simulink library "PQFV_lib"  (Simulink 8.1)
settings: Solver=ode45  StartTime=0.0  StopTime=10.0  RelTol=1e-3
undefined symbols (not defined in the file): Ts
libraries: powerlib_extras x6, RMS_lib x2
settings Model: Creator=RE25624  LastModifiedBy=g73labuser

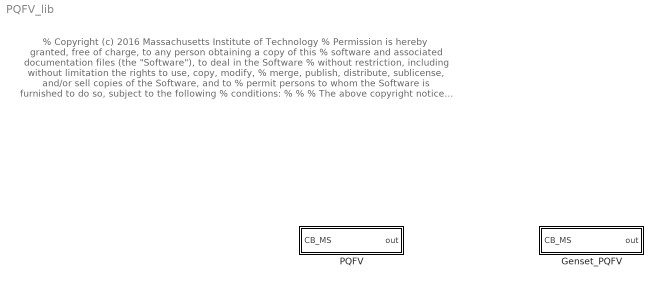
== system PQFV_lib ==
  note: % Copyright (c) 2016 Massachusetts Institute of Technology
      | % Permission is hereby granted, free of charge, to any person obtaining a copy of this
      | % software and associated documentation files (the "Software"), to deal in the Software
      | % without restriction, including without limitation the rights to use, copy, modify,
      | % merge, publish, distribute, sublicense, and/or sell copies of the Software, and to
      | % permit persons to whom the Software is furnished to do so, subject to the following
      | % conditions:
      | %
      | %
      | % The above copyright notice and this permission notice shall be included in
      | % all copies or substantial portions of the Software.
      | %
      | % THE SOFTWARE IS PROVIDED "AS IS", WITHOUT WARRANTY OF ANY KIND, EXPRESS OR IMPLIED,
      | % INCLUDING BUT NOT LIMITED TO THE WARRANTIES OF MERCHANTABILITY, FITNESS FOR A
      | % PARTICULAR PURPOSE AND NONINFRINGEMENT. IN NO EVENT SHALL THE AUTHORS OR COPYRIGHT
      | % HOLDERS BE LIABLE FOR ANY CLAIM, DAMAGES OR OTHER LIABILITY, WHETHER IN AN ACTION
      | % OF CONTRACT, TORT OR OTHERWISE, ARISING FROM, OUT OF OR IN CONNECTION WITH THE
      | % SOFTWARE OR THE USE OR OTHER DEALINGS IN THE SOFTWARE.
      | %
      | %
      | %%
  Genset_PQFV : Subsystem  mask(PQFV){VRMSLL=13800, Ts=Ts}
      mask prompts: VRMSLL "Nominal VRMSLL"; Ts "Sample Time [Sec]"
      mask help:
      | Block inputs: circuit breaker measurements
      | Block outputs: kW, kVAR, Hz, VRMSLL, Vpu, cb-status
      | -voltage as seem at the entry-point of the circuit breaker
  PQFV : Subsystem  mask(PQFV){VRMSLL=13800, Ts=Ts}
      mask prompts: VRMSLL "Nominal VRMSLL"; Ts "Sample Time [Sec]"
      mask help:
      | Block inputs: circuit breaker measurements
      | Block outputs: kW, kVAR, Hz, VRMSLL, Vpu, cb-status
      | -voltage as seem at the entry-point of the circuit breaker

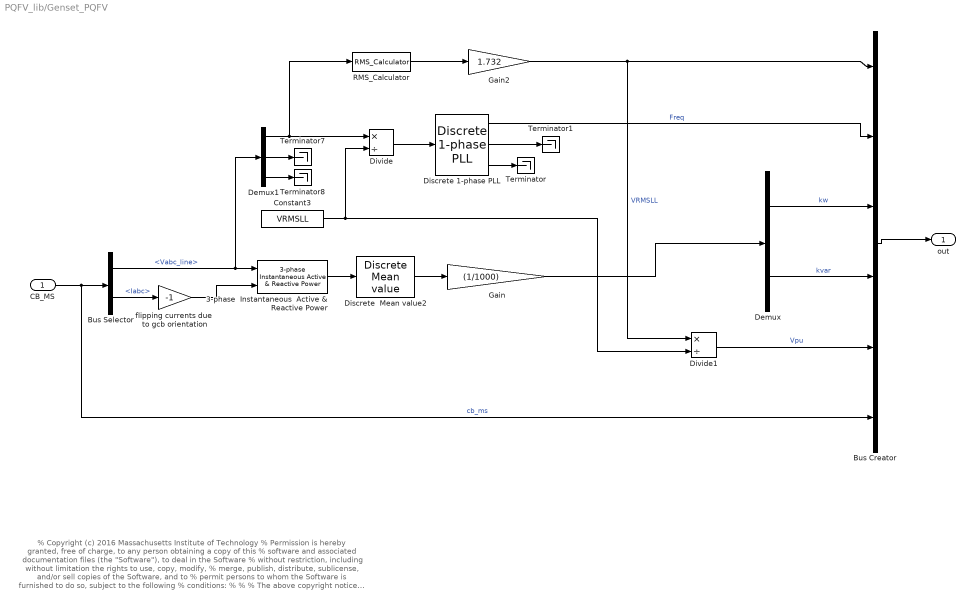
== system PQFV_lib/Genset_PQFV ==
  note: % Copyright (c) 2016 Massachusetts Institute of Technology
      | % Permission is hereby granted, free of charge, to any person obtaining a copy of this
      | % software and associated documentation files (the "Software"), to deal in the Software
      | % without restriction, including without limitation the rights to use, copy, modify,
      | % merge, publish, distribute, sublicense, and/or sell copies of the Software, and to
      | % permit persons to whom the Software is furnished to do so, subject to the following
      | % conditions:
      | %
      | %
      | % The above copyright notice and this permission notice shall be included in
      | % all copies or substantial portions of the Software.
      | %
      | % THE SOFTWARE IS PROVIDED "AS IS", WITHOUT WARRANTY OF ANY KIND, EXPRESS OR IMPLIED,
      | % INCLUDING BUT NOT LIMITED TO THE WARRANTIES OF MERCHANTABILITY, FITNESS FOR A
      | % PARTICULAR PURPOSE AND NONINFRINGEMENT. IN NO EVENT SHALL THE AUTHORS OR COPYRIGHT
      | % HOLDERS BE LIABLE FOR ANY CLAIM, DAMAGES OR OTHER LIABILITY, WHETHER IN AN ACTION
      | % OF CONTRACT, TORT OR OTHERWISE, ARISING FROM, OUT OF OR IN CONNECTION WITH THE
      | % SOFTWARE OR THE USE OR OTHER DEALINGS IN THE SOFTWARE.
      | %
      | %
      | %%
  CB_MS : Inport
  3-phase  Instantaneous  Active & Reactive Power : powerlib_extras/Measurements/3-phase  Instantaneous  Active & Reactive Power
  Bus Creator : BusCreator  Inputs=6
  Bus Selector : BusSelector  OutputSignals=Vabc_line,Iabc
  Constant3 : Constant  Value=VRMSLL
  Demux : Demux  Outputs=2
  Demux1 : Demux  Outputs=3
  Discrete 1-phase PLL : powerlib_extras/Discrete  Control Blocks/Discrete 1-phase PLL  Fmin=45  Par_Init=[0 60]  ParK=[ 180 3200 1]  Ts=Ts  AGC=on
  Discrete  Mean value2 : powerlib_extras/Discrete Measurements/Discrete  Mean value  Freq=60  Vinit=0  Ts=Ts
  Divide : Product  Inputs=*/
  Divide1 : Product  Inputs=*/
  Gain : Gain  Gain=(1/1000)
  Gain2 : Gain  Gain=1.732
  RMS_Calculator : RMS_lib/RMS_Calculator
  Terminator{,1,7..8} (4 alike) : Terminator
  flipping currents due  to gcb orientation : Gain  Gain=-1
  out : Outport
  wires:
  flipping currents due  to gcb orientation/1 -> 3-phase  Instantaneous  Active & Reactive Power/2
  CB_MS/1 -> Bus Selector/1, Bus Creator/6  "cb_ms"
  Divide1/1 -> Bus Creator/5  "Vpu"
  Gain2/1 -> Divide1/1, Bus Creator/1  "VRMSLL"
  Bus Creator/1 -> out/1
  Bus Selector/2 -> flipping currents due  to gcb orientation/1  "<Iabc>"
  Bus Selector/1 -> 3-phase  Instantaneous  Active & Reactive Power/1, Demux1/1  "<Vabc_line>"
  Demux/2 -> Bus Creator/4  "kvar"
  Demux/1 -> Bus Creator/3  "kw"
  Discrete  Mean value2/1 -> Gain/1
  3-phase  Instantaneous  Active & Reactive Power/1 -> Discrete  Mean value2/1
  Gain/1 -> Demux/1
  Discrete 1-phase PLL/1 -> Bus Creator/2  "Freq"
  Discrete 1-phase PLL/3 -> Terminator/1
  Divide/1 -> Discrete 1-phase PLL/1
  Discrete 1-phase PLL/2 -> Terminator1/1
  Demux1/1 -> RMS_Calculator/1, Divide/1
  Demux1/2 -> Terminator7/1
  Demux1/3 -> Terminator8/1
  Constant3/1 -> Divide/2, Divide1/2
  RMS_Calculator/1 -> Gain2/1

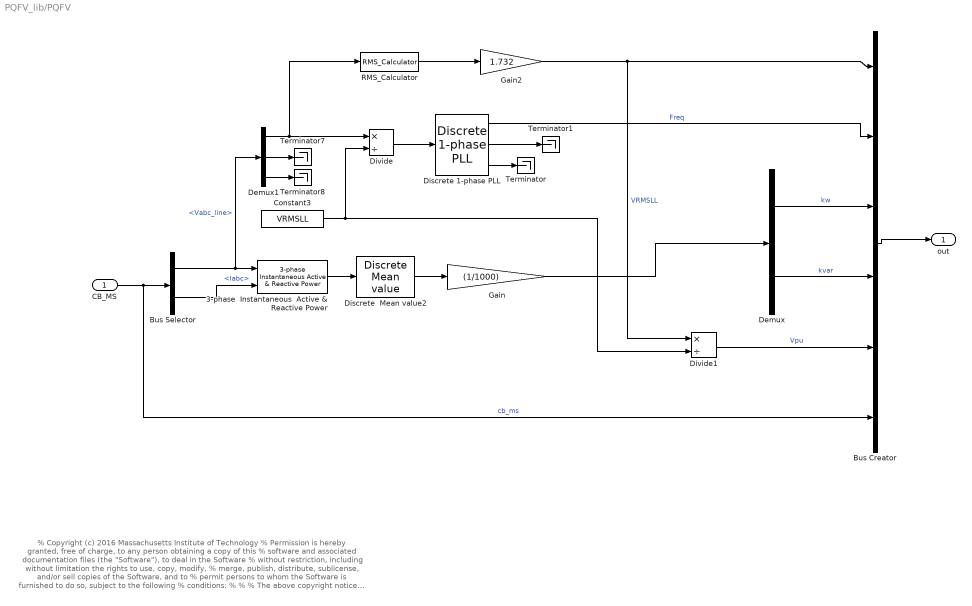
== system PQFV_lib/PQFV ==
  note: % Copyright (c) 2016 Massachusetts Institute of Technology
      | % Permission is hereby granted, free of charge, to any person obtaining a copy of this
      | % software and associated documentation files (the "Software"), to deal in the Software
      | % without restriction, including without limitation the rights to use, copy, modify,
      | % merge, publish, distribute, sublicense, and/or sell copies of the Software, and to
      | % permit persons to whom the Software is furnished to do so, subject to the following
      | % conditions:
      | %
      | %
      | % The above copyright notice and this permission notice shall be included in
      | % all copies or substantial portions of the Software.
      | %
      | % THE SOFTWARE IS PROVIDED "AS IS", WITHOUT WARRANTY OF ANY KIND, EXPRESS OR IMPLIED,
      | % INCLUDING BUT NOT LIMITED TO THE WARRANTIES OF MERCHANTABILITY, FITNESS FOR A
      | % PARTICULAR PURPOSE AND NONINFRINGEMENT. IN NO EVENT SHALL THE AUTHORS OR COPYRIGHT
      | % HOLDERS BE LIABLE FOR ANY CLAIM, DAMAGES OR OTHER LIABILITY, WHETHER IN AN ACTION
      | % OF CONTRACT, TORT OR OTHERWISE, ARISING FROM, OUT OF OR IN CONNECTION WITH THE
      | % SOFTWARE OR THE USE OR OTHER DEALINGS IN THE SOFTWARE.
      | %
      | %
      | %%
  CB_MS : Inport
  3-phase  Instantaneous  Active & Reactive Power : powerlib_extras/Measurements/3-phase  Instantaneous  Active & Reactive Power
  Bus Creator : BusCreator  Inputs=6
  Bus Selector : BusSelector  OutputSignals=Vabc_line,Iabc
  Constant3 : Constant  Value=VRMSLL
  Demux : Demux  Outputs=2
  Demux1 : Demux  Outputs=3
  Discrete 1-phase PLL : powerlib_extras/Discrete  Control Blocks/Discrete 1-phase PLL  Fmin=45  Par_Init=[0 60]  ParK=[ 180 3200 1]  Ts=Ts  AGC=on
  Discrete  Mean value2 : powerlib_extras/Discrete Measurements/Discrete  Mean value  Freq=60  Vinit=0  Ts=Ts
  Divide : Product  Inputs=*/
  Divide1 : Product  Inputs=*/
  Gain : Gain  Gain=(1/1000)
  Gain2 : Gain  Gain=1.732
  RMS_Calculator : RMS_lib/RMS_Calculator  Ts=Ts
  Terminator{,1,7..8} (4 alike) : Terminator
  out : Outport
  wires:
  CB_MS/1 -> Bus Selector/1, Bus Creator/6  "cb_ms"
  Divide1/1 -> Bus Creator/5  "Vpu"
  Gain2/1 -> Divide1/1, Bus Creator/1  "VRMSLL"
  Bus Creator/1 -> out/1
  Bus Selector/2 -> 3-phase  Instantaneous  Active & Reactive Power/2  "<Iabc>"
  Bus Selector/1 -> 3-phase  Instantaneous  Active & Reactive Power/1, Demux1/1  "<Vabc_line>"
  Demux/2 -> Bus Creator/4  "kvar"
  Demux/1 -> Bus Creator/3  "kw"
  Discrete  Mean value2/1 -> Gain/1
  3-phase  Instantaneous  Active & Reactive Power/1 -> Discrete  Mean value2/1
  Gain/1 -> Demux/1
  Discrete 1-phase PLL/1 -> Bus Creator/2  "Freq"
  Discrete 1-phase PLL/3 -> Terminator/1
  Divide/1 -> Discrete 1-phase PLL/1
  Discrete 1-phase PLL/2 -> Terminator1/1
  Demux1/1 -> RMS_Calculator/1, Divide/1
  Demux1/2 -> Terminator7/1
  Demux1/3 -> Terminator8/1
  Constant3/1 -> Divide/2, Divide1/2
  RMS_Calculator/1 -> Gain2/1
